simulink library "BLE_Library"  (R2017b)
settings: Solver=VariableStepAuto  StartTime=0.0  StopTime=10.0  RelTol=1e-3
values from neighbouring files (symbols this model uses):
  D = D/ScaleCoefficient    [BLE_PostLoad.m]    (also in new_BLE_model.m = zeros(N_BLE,N_BLE+1))
undefined symbols (not defined in the file or in its folder): ADV_IND_AccA, ADV_IND_id, BT_Hop_Separation, BT_Samples_Per_Symbol, CONNECT_IND_id, CONNECT_IND_length, F3B672D172DF, F506B10B1B3E, Header, LL_DATA_EMPTY_length, LL_DATA_id, magnitude, Payload, Preamble, Slot_Ts, T_IFS
libraries: BLE_Library x56, simulink x39, commutil2 x29, dspindex x17, commdigbbndfm2 x5, dspsigops x2, commrandsrc3 x2, dspstat3 x2, dspsrcs4 x1, dsparch4 x1, commdigbbndcpm2 x1
(part 5 of 5)

== stateflow chart BLE_Library/BLE slave/Advertising state control chart ==
  settings: executeAtInitialization=1
  state Standby
    en: ChIdx=37; TxEn=false; RxEn=false; SamplEn=false; dt=1;
    RxPDU_type=CONNECT_IND_id; TxPDU_type=ADV_IND_id;
  state AdvertStart
    en: TxEn=true;
    du,ex: tn=tn+1;
  state ReplyScan
  state AdvertEnd
    en: disp(GenMsg(['S',nD,': advertising event closed at'],Dclock*1e3))
  state ConnectionCreated_Receive_end
    en,du,ex:
    T_LLconnSupervision=T_LLconnSupervision+1;
  state CheckAnchor_Receive_start
    en: RxEn=true; ChIdx=getChIdx(lastUnmappedChannel,Hop,ChM); lastUnmappedChannel=ChIdx; connEventCounter=mod(connEventCounter+1,65536);
    du,ex: T_LLconnSupervision=T_LLconnSupervision+1;
  state AnchorPointFailed_Receive_end
    en:RxEn=false;
    disp(GenMsg(['S',nD,': anchor point failed to establish for M',r_m,' at'],Dclock*1e3))
    du,ex: T_LLconnSupervision=T_LLconnSupervision+1;
  state AnchorPointPassed_Receive_continue
    en: T_LLconnSupervision=0; TimeoutBound=Timeout*10e3; k=LL_DATA_EMPTY_length;
    TxPDU_type=LL_DATA_id; RxNewData=true; TxNewData=true; m_MD=1; n_failedMD=0; n_DataPDU=0;
    ex: k=k+1; T_LLconnSupervision=T_LLconnSupervision+1;
  state ConnectionEvent_start_Receive_start
    en: ChIdx=getChIdx(lastUnmappedChannel,Hop,ChM);
    lastUnmappedChannel=ChIdx; RxEn=true; m_MD=1; n_failedMD=0; n_DataPDU=0;
    connEventCounter=mod(connEventCounter+1,65536); k=1;
    du,ex: k=k+1; T_LLconnSupervision=T_LLconnSupervision+1;
  state Receive_start
    en: RxEn=true;
    du,ex: k=k+1; T_LLconnSupervision=T_LLconnSupervision+1;
  state idx=getChIdx(idx_1,didx,chMap) [function]
    (default) -> (junction 326) : {idx=mod(idx_1+didx,37);}
    (junction 326) -> (junction 318) [order 1] : [chMap(idx+1)==1]
    (junction 326) -> (junction 315) [order 2] : {idxRemap=mod(idx,sum(chMap));
        | ind=-1; v=1;}
    (junction 312) -> (junction 327) [order 1] : [chMap(v)==1]{ind=ind+1;}
    (junction 310) -> (junction 312) [order 1] : [v<41]
    (junction 327) -> (junction 307) [order 2]
    (junction 315) -> (junction 310)
    (junction 312) -> (junction 307) [order 2]
    (junction 327) -> (junction 329) [order 1] : [idxRemap==ind]{idx=uint16(v-1);v=40;}
    (junction 307) -> (junction 310) : {v=v+1;}
    (junction 310) -> (junction 313) [order 2]
    (junction 329) -> (junction 307)
  note: NDM=1, when MDbit=1, ensures that device replies
      | to the received packet after 150 us independent of
      | packet loss or CRC match (BLE standard says that two
      | consecutive packets received with an invalid CRC
      | match within a connection event shall close the
      | event). This is needed to ensure higher sampling
      | rates than 133.33 Hz (7.5 ms) in noisy environment.
  state Receive_end_Send_prepare
    du,ex: k=k+1; T_LLconnSupervision=T_LLconnSupervision+1;
  state Send_start
    en: TxEn=true; SamplEn=true;
    du,ex: k=k+1; T_LLconnSupervision=T_LLconnSupervision+1;
  state Send_end
    en: TxEn=false; SamplEn=false;
    du,ex: k=k+1; T_LLconnSupervision=T_LLconnSupervision+1;
  note: Additional condition ensures frequency hopping intervals to conform to the connInterval independent of the received MD value from the master.
  state ConnectionEvent_continue_Receive_prepare
    du,ex: k=k+1; T_LLconnSupervision=T_LLconnSupervision+1;
  state Receive_end_ConnectionEvent_end
    du,ex: T_LLconnSupervision=T_LLconnSupervision+1;
  (default) -> Standby
  (junction 522) -> Standby
  (junction 593) -> (junction 522) : {disp(GenMsg(['S',nD,': connection terminated with M',r_m,' at'],Dclock*1e3))}
  Standby -> (junction 782) : [TurnOn]{disp(GenMsg(['S',nD,': advertising state entered at'],Dclock*1e3))}
  (junction 500) -> (junction 782)
  AdvertEnd -> (junction 500) : after(T_advEvent-tn,tick)
      | {ChIdx=37;}
  (junction 782) -> AdvertStart : {tn=1; advDelay=floor(10001*mod(rand(1,1)*nD,1));
      | T_advEvent=advInterval+advDelay;
      | disp(GenMsg(['S',nD,': advertising event started at'],Dclock*1e3))}
  AdvertStart -> (junction 101) : [after(TXACTIVE(1),tick)]{TxEn=false;}
  (junction 101) -> (junction 103) : after(TXACTIVE(1)+T_IFS+dt,tick){RxEn=true;}
  (junction 7) -> AdvertStart [order 1] : [ChIdx<39]
      | {ChIdx=ChIdx+1;}
  (junction 103) -> (junction 168) : after(TXACTIVE(1)+T_IFS+dt+CONNECT_IND_length,tick){RxEn=false;}
  (junction 33) -> ReplyScan [order 1] : [Reply_scan==1]
  (junction 168) -> (junction 5) [order 3]
  (junction 168) -> (junction 33) [order 2] : [scan_req==1]
  (junction 33) -> (junction 18) [order 2]
  (junction 168) -> (junction 24) [order 1] : [con_req==1]
  (junction 5) -> (junction 58) : after(T_ADV_IND,tick)
  (junction 7) -> AdvertEnd [order 2]
  (junction 58) -> (junction 7)
  (junction 18) -> (junction 58) [order 1] : [Continue_ADV==1]
  (junction 504) -> (junction 7)
  (junction 18) -> (junction 504) [order 2] : {ChIdx=39;}
  (junction 24) -> (junction 18) [order 2]
  (junction 24) -> ConnectionCreated_Receive_end [order 1] : [Reply_connect==1]{
      | SCA=connParam(1);
      | Hop=connParam(2);
      | ChM=connParam(3:42);
      | Timeout=connParam(43);
      | Latency=connParam(44);
      | Interval=connParam(45);
      | WinOffset=connParam(46);
      | WinSize=connParam(47);
      | RxPDU_type=LL_DATA_id;
      | lastUnmappedChannel=0;
      | transmitSeqNum=false;
      | nextExpectedSeqNum=false;
      | MD_SN_NESN_out=[false; false; false];
      | T_LLconnSupervision=0;
      | TimeoutBound=6*Interval*1250;
      | r_m=GenM(GetMInd(master_AdvAs, master_Names, InitA)); disp(GenMsg(['S',nD,': connection created with M',r_m,' at'],Dclock*1e3))}
  ConnectionCreated_Receive_end -> CheckAnchor_Receive_start : [after(1250*(1+WinOffset),tick)]{connEventCounter=0;}
  (junction 591) -> (junction 593) [order 1] : [T_LLconnSupervision>=TimeoutBound]
  (junction 591) -> CheckAnchor_Receive_start [order 2]
  (junction 520) -> (junction 593)
  AnchorPointFailed_Receive_end -> (junction 591) : [after((Interval-WinSize)*1250,tick) || T_LLconnSupervision>=TimeoutBound]
  CheckAnchor_Receive_start -> (junction 357) : [after(WinSize*1250,tick) || setAnchor || T_LLconnSupervision>=TimeoutBound]
  (junction 357) -> AnchorPointFailed_Receive_end [order 3]
  (junction 357) -> AnchorPointPassed_Receive_continue [order 2] : [setAnchor]{disp(GenMsg(['S',nD,': anchor point established for M',r_m,' at'],(Dclock-40*Slot_Ts)*1e3))}
  (junction 357) -> (junction 621) [order 1] : [T_LLconnSupervision>=TimeoutBound]
  AnchorPointPassed_Receive_continue -> (junction 793) : [after(LL_DATA_EMPTY_length-40,tick)]{
      | disp(GenMsg(['S',nD,': connection established with M',r_m,' at'],Dclock*1e3));}
  (junction 621) -> (junction 520)
  (junction 614) -> (junction 621)
  (junction 717) -> ConnectionEvent_start_Receive_start
  ConnectionEvent_start_Receive_start -> (junction 677)
  Receive_start -> (junction 677)
  (junction 677) -> (junction 612) : [after(LL_DATA_EMPTY_length,tick) || T_LLconnSupervision>=TimeoutBound]
  (junction 741) -> Receive_start
  (junction 612) -> (junction 614) [order 1] : [T_LLconnSupervision>=TimeoutBound]
  (junction 793) -> (junction 612)
  (junction 555) -> (junction 614)
  (junction 612) -> (junction 387) [order 2] : {RxEn=false; n_DataPDU=n_DataPDU+1;
      | MD=MD_SN_NESN_in(1); SN=MD_SN_NESN_in(2); NESN=MD_SN_NESN_in(3);
      | [MD_SN_NESN_out(1),m_MD]=SetMD(m_packets, m_MD);}
  (junction 387) -> (junction 390) [order 1] : [CRC_OK_LL_DATA]{n_failedMD=0; T_LLconnSupervision=0;
      | disp(GenMsg(['S',nD,': CRC passed from M',r_m,' at'],Dclock*1e3));}
  (junction 390) -> (junction 391) [order 1] : [SN==nextExpectedSeqNum]{RxNewData=true;
      | nextExpectedSeqNum=not(nextExpectedSeqNum);}
  (junction 390) -> (junction 391) [order 2] : {RxNewData=false;}
  (junction 391) -> (junction 396) [order 2] : {TxNewData=false;}
  (junction 387) -> (junction 667) [order 2] : {n_failedMD=n_failedMD+1;
      | disp(GenMsg(['S',nD,': CRC failed from M',r_m,' at'],Dclock*1e3))}
  (junction 391) -> (junction 396) [order 1] : [NESN~=transmitSeqNum]{TxNewData=true;
      | transmitSeqNum=not(transmitSeqNum);}
  (junction 799) -> (junction 731) [order 1] : [P_En]
  (junction 667) -> (junction 799) [order 1] : [n_DataPDU>1 && ~(NDM && MDbit)]
  (junction 731) -> (junction 806)
  (junction 799) -> (junction 811) [order 2]
  (junction 667) -> Receive_end_Send_prepare [order 2]
  (junction 396) -> Receive_end_Send_prepare : {MD_SN_NESN_out(3)=nextExpectedSeqNum;
      | MD_SN_NESN_out(2)=transmitSeqNum;}
  (junction 806) -> Receive_end_Send_prepare [order 1] : [n_failedMD<2]
  (junction 806) -> (junction 809) [order 2]
  Receive_end_Send_prepare -> (junction 371) : [after(T_IFS-dt,tick) || T_LLconnSupervision>=TimeoutBound]
  (junction 809) -> (junction 811)
  (junction 811) -> Receive_end_ConnectionEvent_end
  (junction 371) -> (junction 555) [order 1] : [T_LLconnSupervision>=TimeoutBound]
  (junction 371) -> Send_start [order 2]
  (junction 708) -> (junction 555)
  Send_start -> (junction 558) : [after(TXACTIVE(2),tick) || T_LLconnSupervision>=TimeoutBound]
  (junction 558) -> (junction 708) [order 1] : [T_LLconnSupervision>=TimeoutBound]
  (junction 558) -> Send_end [order 2]
  (junction 713) -> (junction 708)
  Send_end -> (junction 700)
  (junction 700) -> Receive_end_ConnectionEvent_end [order 2]
  (junction 700) -> ConnectionEvent_continue_Receive_prepare [order 1] : [(MD && Interval*1250-k+1>=3*T_IFS+LL_DATA_EMPTY_length+TXACTIVE(2)) || MD_SN_NESN_out(1)]
  Receive_end_ConnectionEvent_end -> (junction 692) : [after(Interval*1250-k+1,tick) || T_LLconnSupervision>=TimeoutBound]
  ConnectionEvent_continue_Receive_prepare -> (junction 740) : [after(T_IFS-1+dt,tick) || T_LLconnSupervision>=TimeoutBound]
  (junction 692) -> (junction 713) [order 1] : [T_LLconnSupervision>=TimeoutBound]
  (junction 740) -> (junction 692) [order 1] : [T_LLconnSupervision>=TimeoutBound]
  (junction 740) -> (junction 741) [order 2]
  (junction 692) -> (junction 718) [order 2]
  (junction 718) -> (junction 717)
  data: x function_input; m function_output; MasterList function_input; mInd function_output; MasterIdxs function_input; MasterInitA function_input; idx function_output; idx_1 function_input; didx function_input; chMap function_input; m_max function_input; md function_output; m_old function_input; m_new function_output; str function_input; msg function_output; t function_input; ChIdx output uint16; scan_req input; con_req input; Reply_scan input; Reply_connect input; Continue_ADV input; TxEn output; TxPDU_type output; RxEn output; TXACTIVE input; T_IFS parameter; T_ADV_IND parameter; advDelay local; advInterval parameter; T_advEvent local; connParam input; SCA local; Hop local; Latency local; Interval local; WinOffset local; WinSize local; CONNECT_IND_id parameter; RxPDU_type output; LL_DATA_id parameter; lastUnmappedChannel local uint16; ChM local; CONNECT_IND_length parameter; LL_DATA_EMPTY_length parameter; setAnchor input; P_En input; ADV_IND_id parameter; nextExpectedSeqNum local; transmitSeqNum local; MD_SN_NESN_in input boolean; MD local; NESN local; SN local; CRC_OK_LL_DATA input boolean; MD_SN_NESN_out output boolean; TxNewData output; RxNewData output; connEventCounter output; T_LLconnSupervision output; TimeoutBound local; Timeout local; Dclock input; Slot_Ts parameter; TurnOn input; tn local; m_MD local; m_packets parameter; n_failedMD local; k local; SamplEn output boolean; nD parameter; InitA input; master_Names parameter; r_m local; master_AdvAs parameter; dt local; NDM parameter; n_DataPDU local; MDbit parameter
  function m = GenM(x):
    | function m = GenM(x)
    | 
    | coder.extrinsic('sprintf')
    | m = sprintf('%d',x);
  function mInd = GetMInd(MasterList, MasterIdxs, MasterInitA):
    | function mInd = GetMInd(MasterList, MasterIdxs, MasterInitA)
    | 
    | mInd=0;
    | for k=1:size(MasterList,2)
    |     if sum(MasterList(:,k)==MasterInitA)==48
    |         mInd=MasterIdxs(k);
    |         break;
    |     end
    | end
  function [md,m_new] = SetMD(m_max,m_old):
    | function [md,m_new] = SetMD(m_max,m_old)
    | 
    | md=0;
    | 
    | if m_old < m_max
    |     md=1;
    |     m_new=m_old+1;
    | else
    |     m_new=1;
    | end
  function msg = GenMsg(str,t):
    | function msg = GenMsg(str,t)
    | 
    | coder.extrinsic('sprintf')
    | msg = sprintf("%s %0.3f ms",str,t);

== matlab function BLE_Library/BLE slave/Battery Status/MATLAB Function ==
  data: u input; PowerLevel output; PowerEn output boolean; ChargingEn output boolean
function [PowerLevel,PowerEn,ChargingEn] = fcn(u)

if u>=1
    PowerLevel=1;
    ChargingEn=false;
    PowerEn=true;
elseif u<=0
    PowerLevel=0;
    ChargingEn=true;
    PowerEn=false;
else
    PowerLevel=u;
    ChargingEn=true;
    PowerEn=true;
end

== matlab function BLE_Library/BLE slave/Battery Status/Subsystem7/MATLAB Function ==
  data: u input; y output
function y = fcn(u)

if u<=0
    y=0;
elseif u>0&&u<=20
    y=20;
elseif u>20&&u<=40
    y=40;
elseif u>40&&u<=60
    y=60;
elseif u>60&&u<=80
    y=80;
else
    y=100;
end

== matlab function BLE_Library/BLE slave/LL_DATA/MATLAB Function ==
  settings: updateMethod=DISCRETE  sampleTime=Slot_Ts
  data: AccessAddress input boolean size=[32 1]; Preamble output boolean size=[8 1]
function Preamble = fcn(AccessAddress)

if AccessAddress(1)
    Preamble=[true false true false true false true false]';
else
    Preamble=[false true false true false true false true]';
end

== stateflow chart BLE_Library/Demodulation, De-whitening, CRC check, PDU/Access Code check, Payload read enable/Payload read enable ==
  settings: executeAtInitialization=1
  state Payload_Disable
    en: k=0;
  state Payload_Enable
    en,du: k=k+1;
  (default) -> Payload_Disable : {PayloadEn=false;}
  Payload_Enable -> Payload_Disable : [~DataEn || k>N_after-1]
      | {PayloadEn=false;}
  Payload_Disable -> Payload_Enable : [AccA_OK]
      | {PayloadEn=true;}
  data: DataEn input; AccA_OK input; PayloadEn output; k local; N_after parameter

== matlab function BLE_Library/Demodulation, De-whitening, CRC check, PDU/De-whitening, CRC check, Data fields/CRC calculation1/CRC generation ==
  data: bin input; CRC output; LFSR input
function CRC = fcn(bin,LFSR)

CRC=false(24,1);
CRC(1)=xor(bin,LFSR(24));
CRC(2)=xor(LFSR(1),CRC(1));
CRC(3)=LFSR(2);
CRC(4)=xor(LFSR(3),CRC(1));
CRC(5)=xor(LFSR(4),CRC(1));
CRC(6)=LFSR(5);
CRC(7)=xor(LFSR(6),CRC(1));
CRC(8:9)=LFSR(7:8);
CRC(10)=xor(LFSR(9),CRC(1));
CRC(11)=xor(LFSR(10),CRC(1));
CRC(12:24)=LFSR(11:23);

== matlab function BLE_Library/Demodulation, De-whitening, CRC check, PDU/De-whitening, CRC check, Data fields/De-whitening/De-whitening ==
  settings: updateMethod=DISCRETE  sampleTime=Slot_Ts
  data: bin input; bout output; LFSR input; LFSR_new output
function [bout,LFSR_new] = fcn(bin,LFSR)

bout=true;
bout(1)=xor(bin,LFSR(7));

LFSR_new=false(7,1);
LFSR_new(1)=LFSR(7);
LFSR_new(2)=LFSR(1);
LFSR_new(3)=LFSR(2);
LFSR_new(4)=LFSR(3);
LFSR_new(5)=xor(LFSR(4),LFSR(7));
LFSR_new(6)=LFSR(5);
LFSR_new(7)=LFSR(6);

== matlab function BLE_Library/Demodulation, De-whitening, CRC check, PDU/De-whitening, CRC check, Data fields/De-whitening/Subsystem/Initial LFSR generation ==
  settings: updateMethod=DISCRETE  sampleTime=Slot_Ts
  data: ChIdx input; LFSR output boolean
function LFSR = fcn(ChIdx)

% ChIdx -- channel index for initial LFR value

LFSR=true(7,1);

a=ChIdx; %dec2bin convertion
oki=zeros(1,6);
for k=1:6
    if a~=0
        oki(k)=rem(a,2);
        a=fix(a/2);
    else
        break;
    end
end
a=flip(oki);
LFSR(2:7)=a>0;
